simulink model "gm_test_min_cost_function_without_delays"  (R2022a)
settings: Solver=FixedStepDiscrete  StartTime=0.0  StopTime=10.0  RelTol=1e-3
undefined symbols (not defined in the file or in its folder): f_c
libraries: hdlmdlgenlib x80
(part 1 of 3)
settings Model: Creator=Andre Merx  LastModifiedBy=Andre Merx
settings SolverCC: AlgebraicLoopSolver=TrustRegion
settings DataIOCC: LimitDataPoints=on  SaveOutput=off  SaveTime=off
settings OptimizationCC: BlockReduction=off  ConditionallyExecuteInputs=off  DefaultParameterBehavior=Inlined  LifeSpan=inf
settings DebuggingCC: AlgebraicLoopMsg=error  InheritedTsInSrcMsg=none  SingleTaskRateTransMsg=error  UnconnectedInputMsg=warning  UnconnectedOutputMsg=warning  UnconnectedLineMsg=warning  AllowSymbolicDim=off  StrictBusMsg=ErrorOnBusTreatedAsVector  SFUnexpectedBacktrackingDiag=warning  SFNoUnconditionalDefaultTransitionDiag=warning  SFExecutionAtInitializationDiag=none  SFMachineParentedDataDiag=warning  ArithmeticOperatorsInVariantConditions=warning
settings HardwareCC: ProdBitPerPointer=32  ProdBitPerSizeT=32  ProdBitPerPtrDiffT=32  ProdLargestAtomicFloat=None  ProdIntDivRoundTo=Undefined  ProdEndianess=Unspecified  ProdWordSize=32  ProdHWDeviceType=ASIC/FPGA->ASIC/FPGA  ProdEqTarget=off
settings SFSimCC: SimUseLocalCustomCode=off  CustomCodeUndefinedFunction=UseInterfaceOnly
settings RTWCC: RTWUseLocalCustomCode=off
settings CodeAppCC: StateflowObjectComments=on
settings GRTTargetCC: TargetLangStandard=C89/C90 (ANSI)
settings ConfigComp: CovScope=ReferencedModels  CovMetricSettings=dw  CovSaveCumulativeToWorkspaceVar=on  CovSaveSingleToWorkspaceVar=on  CovExternalEMLEnable=off  CovSFcnEnable=off

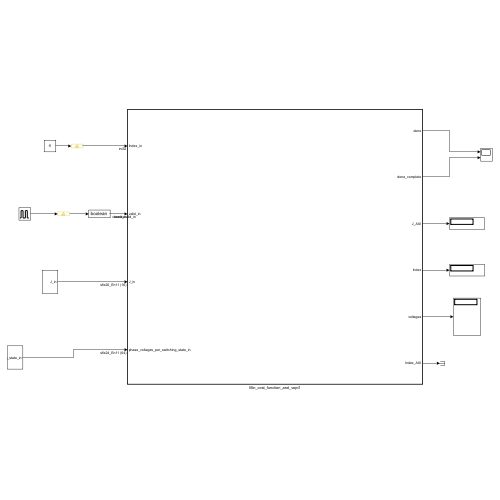
[thumbnail: Simulink's stored preview of the top-level diagram]
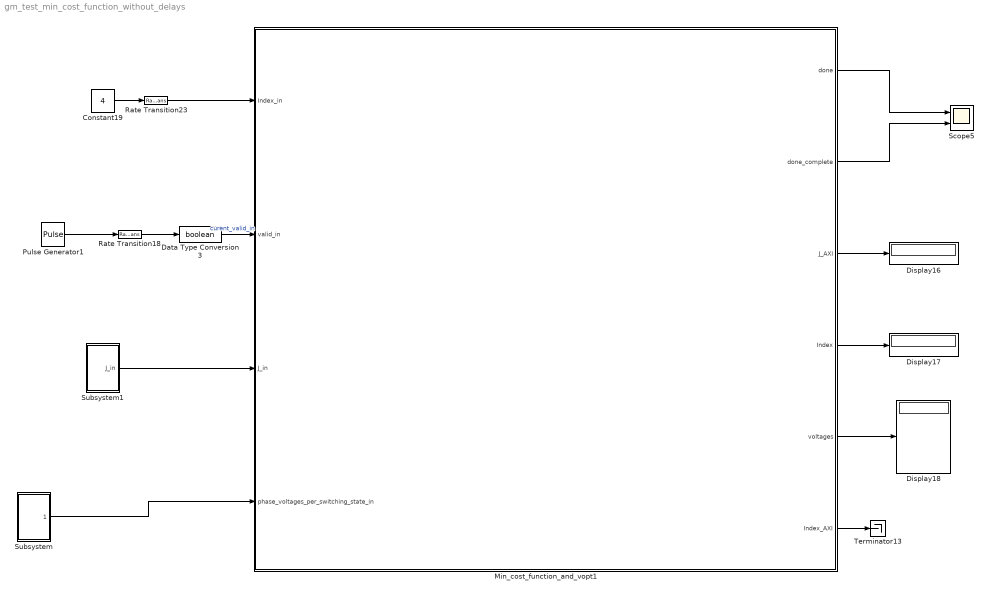
== system gm_test_min_cost_function_without_delays ==
  Constant19 : Constant  Value=4  OutDataTypeStr=int32  SampleTime=-1
  Data Type Conversion3 : DataTypeConversion  OutDataTypeStr=boolean  SaturateOnIntegerOverflow=off  RndMeth=Floor
  Display16 : Display
  Display17 : Display
  Display18 : Display
  Min_cost_function_and_vopt1 : Subsystem  TreatAsAtomicUnit=on
  Pulse Generator1 : DiscretePulseGenerator  PulseType=Time based  Period=1/f_c
  Rate Transition18 : RateTransition  OutPortSampleTime=Rt
  Rate Transition23 : RateTransition  OutPortSampleTime=Rt
  Scope5 : Scope  NumInputPorts=2
  Subsystem : Subsystem
  Subsystem1 : Subsystem
  Terminator13 : Terminator
  wires:
  Constant19/1 -> Rate Transition23/1
  Rate Transition18/1 -> Data Type Conversion3/1
  Pulse Generator1/1 -> Rate Transition18/1
  Data Type Conversion3/1 -> Min_cost_function_and_vopt1/2(valid_in)  "curent_valid_in"
  Rate Transition23/1 -> Min_cost_function_and_vopt1/1(Index_in)
  Min_cost_function_and_vopt1/4(Index) -> Display17/1
  Min_cost_function_and_vopt1/6(Index_AXI) -> Terminator13/1
  Min_cost_function_and_vopt1/1(done) -> Scope5/1
  Min_cost_function_and_vopt1/5(voltages) -> Display18/1
  Min_cost_function_and_vopt1/3(J_AXI) -> Display16/1
  Min_cost_function_and_vopt1/2(done_complete) -> Scope5/2
  Subsystem1/1(J_in) -> Min_cost_function_and_vopt1/3(J_in)
  Subsystem/1(phase_voltages_per_switching_state_in) -> Min_cost_function_and_vopt1/4(phase_voltages_per_switching_state_in)
